simulink model "Test_Copter"  (Simulink 7.4)
settings: Solver=ode45  StartTime=0.0  StopTime=10.0  RelTol=1e-3
libraries: Copter_Library x1
settings Model: Creator=robert  LastModifiedBy=robert

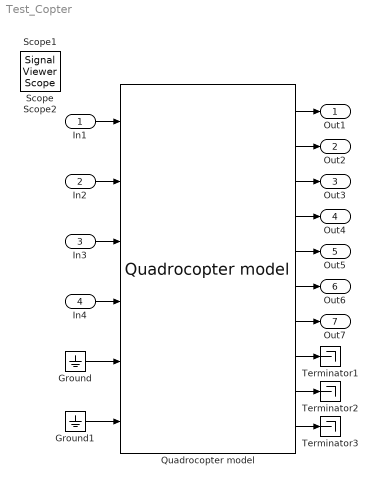
== system Test_Copter ==
  In1 : Inport  OutDataType=fixdt(1, 16)  OutScaling=2^0
  In2 : Inport  Port=2  OutDataType=fixdt(1, 16)  OutScaling=2^0
  In3 : Inport  Port=3  OutDataType=fixdt(1, 16)  OutScaling=2^0
  In4 : Inport  Port=4  OutDataType=fixdt(1, 16)  OutScaling=2^0
  Ground : Ground
  Ground1 : Ground
  Quadrocopter model : Copter_Library/Quadrocopter model  SystemSampleTime=-1
  Terminator1 : Terminator
  Terminator2 : Terminator
  Terminator3 : Terminator
  Out1 : Outport  OutDataType=fixdt(1, 16)  OutScaling=2^0
  Out2 : Outport  Port=2  OutDataType=fixdt(1, 16)  OutScaling=2^0
  Out3 : Outport  Port=3  OutDataType=fixdt(1, 16)  OutScaling=2^0
  Out4 : Outport  Port=4  OutDataType=fixdt(1, 16)  OutScaling=2^0
  Out5 : Outport  Port=5  OutDataType=fixdt(1, 16)  OutScaling=2^0
  Out6 : Outport  Port=6  OutDataType=fixdt(1, 16)  OutScaling=2^0
  Out7 : Outport  Port=7  OutDataType=fixdt(1, 16)  OutScaling=2^0
  Scope : SignalViewerScope  IOType=viewer  RefreshTime=0.035000
      settings: ShowLegends=on
  Scope1 : SignalViewerScope  IOType=viewer  RefreshTime=0.035000
      settings: ShowLegends=on
  Scope2 : SignalViewerScope  IOType=viewer  RefreshTime=0.035000
      settings: ShowLegends=on  SaveName=ScopeData2
  wires:
  Quadrocopter model/7 -> Out7/1
  Quadrocopter model/8 -> Terminator1/1
  Quadrocopter model/9 -> Terminator2/1
  Quadrocopter model/10 -> Terminator3/1
  Ground1/1 -> Quadrocopter model/6
  Ground/1 -> Quadrocopter model/5
  In1/1 -> Quadrocopter model/1
  In2/1 -> Quadrocopter model/2
  In3/1 -> Quadrocopter model/3
  In4/1 -> Quadrocopter model/4
  Quadrocopter model/1 -> Out1/1
  Quadrocopter model/2 -> Out2/1
  Quadrocopter model/3 -> Out3/1
  Quadrocopter model/4 -> Out4/1
  Quadrocopter model/5 -> Out5/1
  Quadrocopter model/6 -> Out6/1
